simulink model "simulation_lab12"  (R2020a)
settings: Solver=VariableStepAuto  StartTime=0.0  StopTime=2  RelTol=1e-3
values from neighbouring files (symbols this model uses):
  Fs = 250    [PS_Lab10.m]    (also in PS_Lab11_datos.mat = 8192)
undefined symbols (not defined in the file or in its folder): D2
settings Model: Creator=DELL  LastModifiedBy=DELL

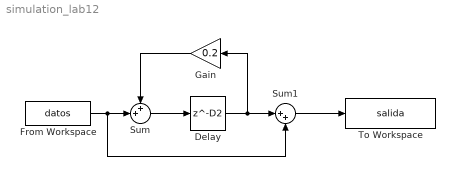
== system simulation_lab12 ==
  Delay : Delay  DelayLength=D2  InitialCondition=0
  From Workspace : FromWorkspace  VariableName=datos  SampleTime=1/Fs  OutputAfterFinalValue=Setting to zero
  Gain : Gain  Gain=0.2
  Sum : Sum  Inputs=++|
  Sum1 : Sum  Inputs=|++
  To Workspace : ToWorkspace  VariableName=salida  SampleTime=-1
  wires:
  From Workspace/1 -> Sum/2, Sum1/2
  Sum/1 -> Delay/1
  Delay/1 -> Gain/1, Sum1/1
  Sum1/1 -> To Workspace/1
  Gain/1 -> Sum/1
